simulink model "LAB1schm"  (R2016a)
settings: Solver=VariableStepAuto  StartTime=0.0  StopTime=10.0  RelTol=1e-3
settings Model: Creator=Григорий  LastModifiedBy=Григорий

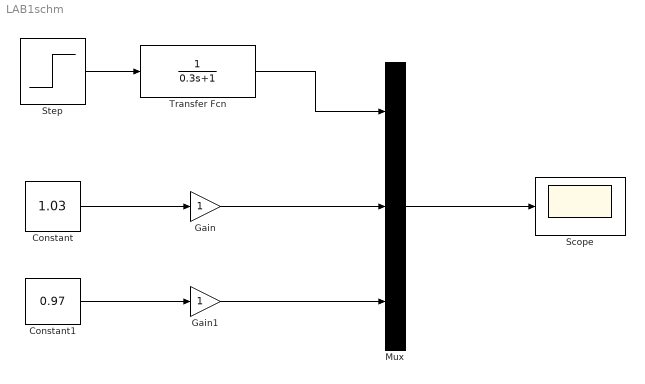
== system LAB1schm ==
  Constant : Constant  Value=1.03
  Constant1 : Constant  Value=0.97
  Gain : Gain
  Gain1 : Gain
  Mux : Mux  Inputs=3
  Scope : Scope
  Step : Step  SampleTime=0
  Transfer Fcn : TransferFcn  Denominator=[0.3 1]
  wires:
  Step/1 -> Transfer Fcn/1
  Mux/1 -> Scope/1
  Transfer Fcn/1 -> Mux/1
  Constant/1 -> Gain/1
  Gain/1 -> Mux/2
  Constant1/1 -> Gain1/1
  Gain1/1 -> Mux/3
